simulink library "actuatorForces"  (R2018b)
settings: Solver=VariableStepAuto  StartTime=0.0  StopTime=10.0  RelTol=1e-3
values from neighbouring files (symbols this model uses):
  b = zeta*(2*sqrt(k*ms))    [Platform.m]    (also in sprungODE.m = system_param.b)
  k = E*A/lus    (= 34906585039.9)    [Platform.m]    (also in sprungODE.m = system_param.k)
undefined symbols (not defined in the file or in its folder): unstretchedL
settings Model: Creator=embeato2  LastModifiedBy=embeato2

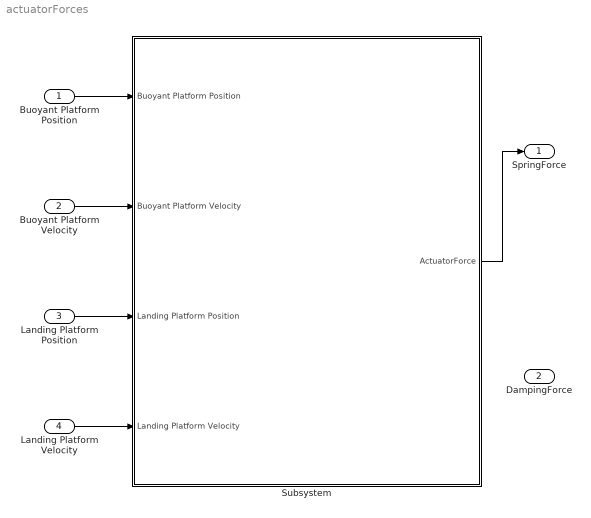
== system actuatorForces ==
  Buoyant Platform Position : Inport
  Buoyant Platform Velocity : Inport  Port=2
  Landing Platform Position : Inport  Port=3
  Landing Platform Velocity : Inport  Port=4
  Subsystem : Subsystem
  SpringForce : Outport
  DampingForce : Outport  Port=2
  wires:
  Buoyant Platform Position/1 -> Subsystem/1(Buoyant Platform Position)
  Buoyant Platform Velocity/1 -> Subsystem/2(Buoyant Platform Velocity)
  Landing Platform Position/1 -> Subsystem/3(Landing Platform Position)
  Landing Platform Velocity/1 -> Subsystem/4(Landing Platform Velocity)
  Subsystem/1(ActuatorForce) -> SpringForce/1
  ? -> DampingForce/1

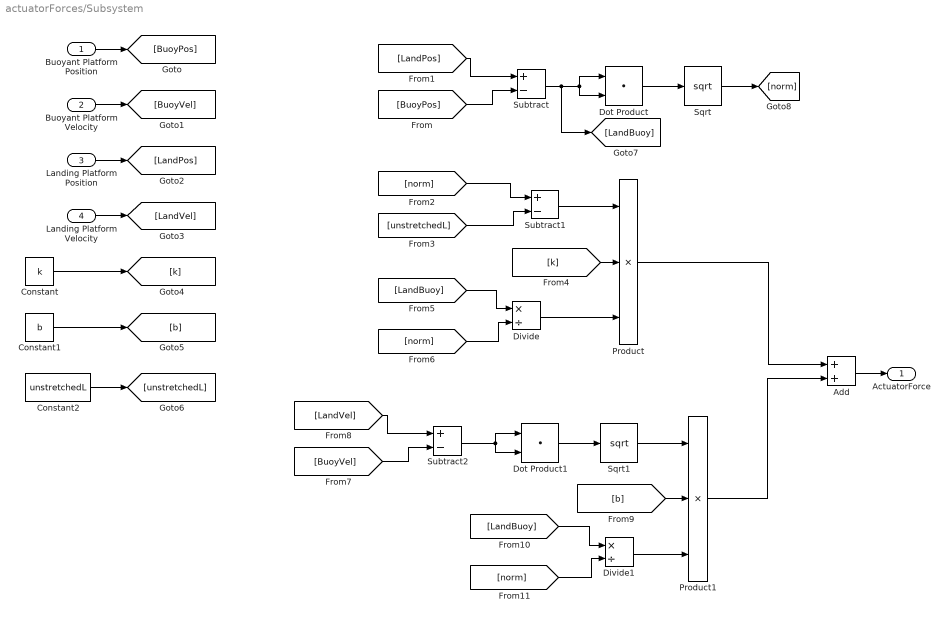
== system actuatorForces/Subsystem ==
  Buoyant Platform Position : Inport
  Buoyant Platform Velocity : Inport  Port=2
  Landing Platform Position : Inport  Port=3
  Landing Platform Velocity : Inport  Port=4
  Add : Sum
  Constant : Constant  Value=k
  Constant1 : Constant  Value=b
  Constant2 : Constant  Value=unstretchedL
  Divide : Product  Inputs=*/
  Divide1 : Product  Inputs=*/
  Dot Product : DotProduct  InputSameDT=on  OutDataTypeStr=Inherit: Inherit via internal rule
  Dot Product1 : DotProduct  InputSameDT=on  OutDataTypeStr=Inherit: Inherit via internal rule
  Product : Product  Inputs=3
  Product1 : Product  Inputs=3
  Sqrt : Sqrt  SaturateOnIntegerOverflow=on
  Sqrt1 : Sqrt  SaturateOnIntegerOverflow=on
  Subtract : Sum  Inputs=+-
  Subtract1 : Sum  Inputs=+-
  Subtract2 : Sum  Inputs=+-
  ActuatorForce : Outport
  wires:
  [LandBuoy] -> Divide/1
  [LandPos] -> Subtract/1
  [k] -> Product/2
  [b] -> Product1/2
  [norm] -> Divide/2
  Constant2/1 -> [unstretchedL]
  [norm] -> Divide1/2
  Buoyant Platform Position/1 -> [BuoyPos]
  Buoyant Platform Velocity/1 -> [BuoyVel]
  Landing Platform Position/1 -> [LandPos]
  [LandVel] -> Subtract2/1
  Landing Platform Velocity/1 -> [LandVel]
  [LandBuoy] -> Divide1/1
  Divide1/1 -> Product1/3
  Constant1/1 -> [b]
  Constant/1 -> [k]
  Product1/1 -> Add/2
  Subtract/1 -> [LandBuoy], Dot Product/1, Dot Product/2
  Dot Product1/1 -> Sqrt1/1
  Sqrt/1 -> [norm]
  [norm] -> Subtract1/1
  Divide/1 -> Product/3
  [BuoyPos] -> Subtract/2
  Dot Product/1 -> Sqrt/1
  [unstretchedL] -> Subtract1/2
  Subtract1/1 -> Product/1
  Subtract2/1 -> Dot Product1/1, Dot Product1/2
  Sqrt1/1 -> Product1/1
  [BuoyVel] -> Subtract2/2
  Add/1 -> ActuatorForce/1
  Product/1 -> Add/1
